simulink model "SIRmodel"  (R2020a)
settings: Solver=VariableStepAuto  StartTime=0.0  StopTime=100  MaxStep=0.01  RelTol=1e-3
values from neighbouring files (symbols this model uses):
  beta = X(1)    [ErroQuadratico.m]    (also in ErroQuadraticoSIR.m)
  I0 = 2    [ErroQuadratico.m]    (also in ErroQuadraticoSIR.m)
  N = 60e6    (= 60000000)    [ErroQuadratico.m]    (also in ErroQuadraticoSIR.m)
  r = X(2)    [ErroQuadratico.m]    (also in ErroQuadraticoSIR.m)
  R0 = 0    [ErroQuadratico.m]    (also in ErroQuadraticoSIR.m)
  S0 = 60e6    (= 60000000)    [ErroQuadratico.m]    (also in ErroQuadraticoSIR.m)
settings Model: Creator=a1  LastModifiedBy=a1

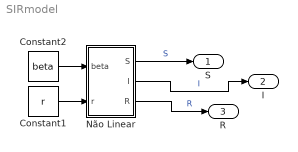
== system SIRmodel ==
  Constant1 : Constant  Value=r
  Constant2 : Constant  Value=beta
  Não Linear : Subsystem
  S : Outport
  I : Outport  Port=2
  R : Outport  Port=3
  wires:
  Constant1/1 -> Não Linear/2(r)
  Não Linear/2(I) -> I/1  "I"
  Não Linear/1(S) -> S/1  "S"
  Não Linear/3(R) -> R/1  "R"
  Constant2/1 -> Não Linear/1(beta)

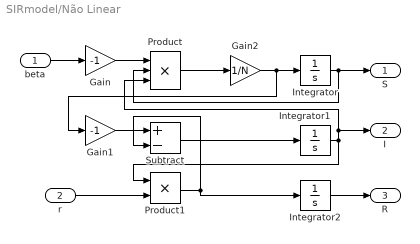
== system SIRmodel/Não Linear ==
  beta : Inport
  r : Inport  Port=2
  Gain : Gain  Gain=-1
  Gain1 : Gain  Gain=-1
  Gain2 : Gain  Gain=1/N
  Integrator : Integrator  InitialCondition=S0
  Integrator1 : Integrator  InitialCondition=I0
  Integrator2 : Integrator  InitialCondition=R0
  Product : Product  Inputs=3
  Product1 : Product
  Subtract : Sum  Inputs=+-
  S : Outport
  I : Outport  Port=2
  R : Outport  Port=3
  wires:
  beta/1 -> Gain/1
  Gain1/1 -> Subtract/1
  Integrator2/1 -> R/1
  Gain/1 -> Product/1
  Product1/1 -> Integrator2/1, Subtract/2
  Product/1 -> Gain2/1
  r/1 -> Product1/2
  Integrator/1 -> S/1, Product/2
  Integrator1/1 -> Product/3, I/1, Product1/1
  Gain2/1 -> Gain1/1, Integrator/1
  Subtract/1 -> Integrator1/1
